simulink model "speed"  (R2014a)
settings: Solver=ode5  StartTime=0.0  StopTime=inf  FixedStep=0.0001  RelTol=1e-3
libraries: dspswit3 x2, dspsigops x2, xpcnilib x1
settings Model: SimulationMode=external  BufferReuse=off  Creator=Lab322  LastModifiedBy=Lab322
settings SolverCC: EnableConcurrentExecution=on
settings OptimizationCC: BlockReduction=off  OptimizeBlockIOStorage=off  BufferReuse=off  GlobalBufferReuse=off  ExpressionFolding=off  LocalBlockOutputs=off
settings HardwareCC: ProdIntDivRoundTo=Zero  ProdEndianess=LittleEndian  ProdHWDeviceType=Generic->32-bit x86 compatible
settings RTWCC: SystemTargetFile=slrt.tlc  TemplateMakefile=slrt_default_tmf  Description=Simulink Real-Time  ProcessScript=slrt_make_rtw_hook  RTWCompilerOptimization=On
settings SimulinkRealTimeCC: GeneratePreprocessorConditionals=Disable all  EnableShiftOperators=on

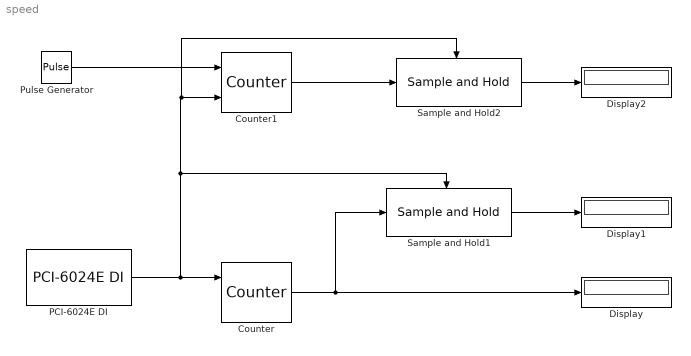
== system speed ==
  Counter : dspswit3/Counter  Direction=Up  CountEvent=Rising edge  CounterSize=User defined  MaxCount=10000000  InitialCount=0  Output=Count  HitValue=32  ResetInput=on  SamplesPerFrame=1  Ts=1  CntDtype=double  HitDtype=Logical
  Counter1 : dspswit3/Counter  Direction=Up  CountEvent=Rising edge  CounterSize=User defined  MaxCount=10000000  InitialCount=0  Output=Count  HitValue=32  ResetInput=on  SamplesPerFrame=1  Ts=1  CntDtype=double  HitDtype=Logical
  Display : Display
  Display1 : Display
  Display2 : Display
  PCI-6024E DI : xpcnilib/Digital Input/E Series/PCI-6024E DI  channel=[7]  sampletime=0.0001  slot=-1
  Pulse Generator : DiscretePulseGenerator  PulseType=Time based  Period=0.001  PulseWidth=50
  Sample and Hold1 : dspsigops/Sample and Hold  trig=Rising edge  initCond=0  latchinput=on
  Sample and Hold2 : dspsigops/Sample and Hold  trig=Rising edge  initCond=0  latchinput=on
  wires:
  PCI-6024E DI/1 -> Sample and Hold1/Trigger, Sample and Hold2/Trigger, Counter1/2, Counter/1
  Counter/1 -> Sample and Hold1/1, Display/1
  Pulse Generator/1 -> Counter1/1
  Sample and Hold1/1 -> Display1/1
  Counter1/1 -> Sample and Hold2/1
  Sample and Hold2/1 -> Display2/1
